simulink model "real_fuzzy"  (R2014b)
settings: Solver=ode4  StartTime=0.0  StopTime=inf  FixedStep=0.001  RelTol=1e-3
undefined symbols (not defined in the file or in its folder): Advantech, PCI, test
libraries: rtwinlib x2, fuzblock x1
settings Model: SimulationMode=external  ExtModeTrigDuration=200000  Creator=Administrator  LastModifiedBy=nk
settings DataIOCC: SignalLoggingSaveFormat=ModelDataLogs
settings OptimizationCC: ExpressionDepthLimit=2147483647  InitFltsAndDblsToZero=on
settings DebuggingCC: SaveWithParameterizedLinksMsg=none  UnderspecifiedInitializationDetection=Classic  MergeDetectMultiDrivingBlocksExec=none  SignalResolutionControl=TryResolveAllWithWarning  MultiTaskDSMMsg=warning  MultiTaskCondExecSysMsg=none  FcnCallInpInsideContextMsg=UseLocalSettings  StateNameClashWarn=warning
settings RTWCC: SystemTargetFile=rtwin.tlc  TemplateMakefile=rtwin.tmf  Description=Real-Time Windows Target  ProcessScript=rtwin_make_rtw_hook  IncludeERTFirstTime=on
settings RTWinTargetCC: TargetFcnLib=ansi_tfl_tmw.mat  TargetLibSuffix=_rtwin.lib  TargetPreCompLibLocation=C:\Program Files\MATLAB\R2014b\toolbox\rtw\targets\rtwin\lib\win64  ModelReferenceCompliant=off  CompOptLevelCompliant=off

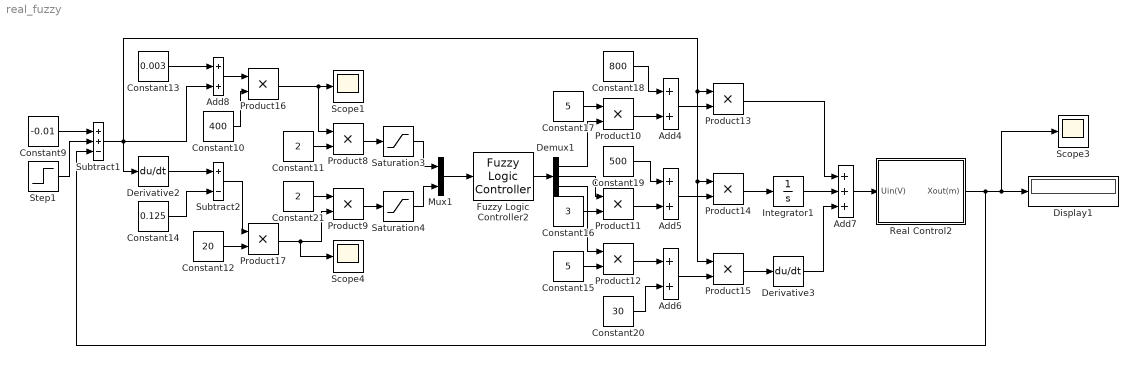
== system real_fuzzy ==
  Add{4..6,8} (4 alike) : Sum
  Add7 : Sum  Inputs=+++
  Constant10 : Constant  Value=400
  Constant11 : Constant  Value=2
  Constant12 : Constant  Value=20
  Constant13 : Constant  Value=0.003
  Constant14 : Constant  Value=0.125
  Constant15 : Constant  Value=5
  Constant16 : Constant  Value=3
  Constant17 : Constant  Value=5
  Constant18 : Constant  Value=800
  Constant19 : Constant  Value=500
  Constant20 : Constant  Value=30
  Constant21 : Constant  Value=2
  Constant9 : Constant  Value=-0.01
  Demux1 : Demux  Outputs=3
  Derivative2 : Derivative
  Derivative3 : Derivative
  Display1 : Display
  Fuzzy Logic Controller2 : fuzblock/Fuzzy Logic  Controller  fis=[test]
  Integrator1 : Integrator
  Mux1 : Mux  Inputs=2
  Product{8..17} (10 alike) : Product
  Real Control2 : Subsystem
  Saturation3 : Saturate
  Saturation4 : Saturate
  Scope1 : Scope
      settings: YMin=-0.012  YMax=-0.007
  Scope3 : Scope
      settings: YMin=-0.01  YMax=-0.0075  SaveName=ScopeData3
  Scope4 : Scope
      settings: TimeRange=1.368821292775666  YMin=-0.007921875000000002  YMax=-0.007546875000000002
  Step1 : Step  Time=10  After=0.001  SampleTime=0
  Subtract1 : Sum  Inputs=++-
  Subtract2 : Sum  Inputs=+-
  wires:
  Subtract1/1 -> Product13/1, Product15/1, Product14/1, Add8/2, Derivative2/1
  Mux1/1 -> Fuzzy Logic Controller2/1
  Fuzzy Logic Controller2/1 -> Demux1/1
  Demux1/1 -> Product10/2
  Demux1/2 -> Product11/1
  Demux1/3 -> Product12/1
  Constant17/1 -> Product10/1
  Constant16/1 -> Product11/2
  Constant15/1 -> Product12/2
  Product10/1 -> Add4/2
  Constant18/1 -> Add4/1
  Product11/1 -> Add5/2
  Constant19/1 -> Add5/1
  Product12/1 -> Add6/1
  Constant20/1 -> Add6/2
  Add4/1 -> Product13/2
  Add5/1 -> Product14/2
  Add6/1 -> Product15/2
  Product15/1 -> Derivative3/1
  Product14/1 -> Integrator1/1
  Product13/1 -> Add7/1
  Integrator1/1 -> Add7/2
  Derivative3/1 -> Add7/3
  Add7/1 -> Real Control2/1(Uin(V))
  Real Control2/1(Xout(m)) -> Display1/1, Scope3/1, Subtract1/3
  Step1/1 -> Subtract1/2
  Constant9/1 -> Subtract1/1
  Saturation4/1 -> Mux1/2
  Saturation3/1 -> Mux1/1
  Product8/1 -> Saturation3/1
  Product9/1 -> Saturation4/1
  Constant21/1 -> Product9/1
  Constant11/1 -> Product8/2
  Product17/1 -> Product9/2, Scope4/1
  Product16/1 -> Product8/1, Scope1/1
  Constant12/1 -> Product17/2
  Constant14/1 -> Subtract2/2
  Derivative2/1 -> Subtract2/1
  Subtract2/1 -> Product17/1
  Add8/1 -> Product16/1
  Constant10/1 -> Product16/2
  Constant13/1 -> Add8/1

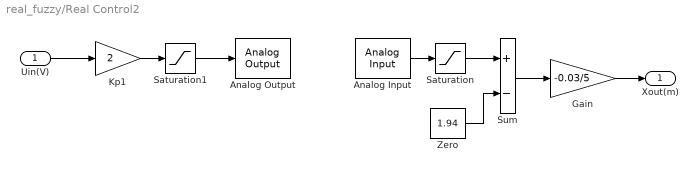
== system real_fuzzy/Real Control2 ==
  Uin(V) : Inport
  Analog Input : rtwinlib/Analog Input  SampleTime=0.001  MaxMissedTicks=10  ShowMissedTicks=off  YieldWhenWaiting=off  DrvName=Advantech/PCI-1711  DrvAddress=4294967295  DrvOptions=zeros(1,0)  Channels=1  RangeMode=1  VoltRange=2  DataType=1
      settings: AttributesFormatString=Advantech\nPCI-1711 [auto]
  Analog Output : rtwinlib/Analog Output  SampleTime=0.001  MaxMissedTicks=10  ShowMissedTicks=off  YieldWhenWaiting=off  DrvName=Advantech/PCI-1711  DrvAddress=4294967295  DrvOptions=zeros(1,0)  Channels=1  RangeMode=1  VoltRange=2  InitialValue=-10  FinalValue=-10
      settings: AttributesFormatString=Advantech\nPCI-1711 [auto]
  Gain : Gain  Gain=-0.03/5  SaturateOnIntegerOverflow=on  OutDataTypeStr=Inherit: Same as input  ParamDataTypeStr=Inherit: Same as input
  Kp1 : Gain  Gain=2  SaturateOnIntegerOverflow=on  OutDataTypeStr=Inherit: Same as input  ParamDataTypeStr=Inherit: Same as input
  Saturation : Saturate  UpperLimit=5  LowerLimit=0
  Saturation1 : Saturate  UpperLimit=10  LowerLimit=0
  Sum : Sum  Inputs=+-  SaturateOnIntegerOverflow=on  OutDataTypeStr=Inherit: Same as first input
  Zero : Constant  Value=1.94  SampleTime=-1
  Xout(m) : Outport
  wires:
  Gain/1 -> Xout(m)/1
  Zero/1 -> Sum/2
  Sum/1 -> Gain/1
  Saturation/1 -> Sum/1
  Analog Input/1 -> Saturation/1
  Kp1/1 -> Saturation1/1
  Uin(V)/1 -> Kp1/1
  Saturation1/1 -> Analog Output/1
